simulink model "pwm_controlled_system"  (R2017a)
settings: Solver=FixedStepAuto  StartTime=0.0  StopTime=t_f  FixedStep=1e-6  RelTol=1e-3
values from neighbouring files (symbols this model uses):
  C_ = C    [load_delay.m]
  Ctilde = [Ctilde, zeros(n_Ctilde, s_nds_i + s_nds_o)]    [load_delay.m]    (also in load_pwm_delayed_controller.m = Ctilde(1, 1:2); load_pwm_delayed_pred_controller.m = Ctilde(1, 1:2); load_pwm_pred_controller.m = Ctilde(1:2))
  x0 = [0; 0]    [sim_controlled_system.m]
undefined symbols (not defined in the file or in its folder): A, B, torque_ref, Tpwm_val, Ts_val, Vcc_val
settings Model: Creator=brunolnetto  LastModifiedBy=brunolnetto
settings SolverCC: AlgebraicLoopSolver=LineSearch

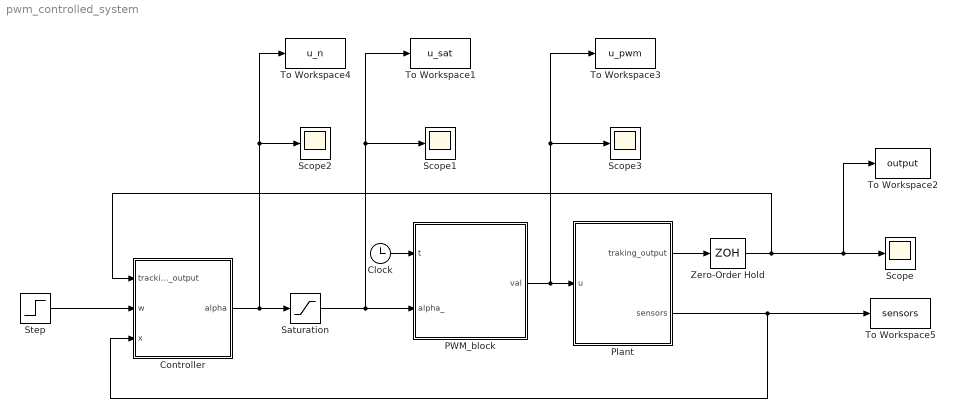
== system pwm_controlled_system ==
  Clock : Clock
  Controller : Subsystem
  PWM_block : MATLAB Function  TreatAsAtomicUnit=on
  Plant : Subsystem
  Saturation : Saturate  UpperLimit=1  LowerLimit=-1
  Scope{,1..3} (4 alike) : Scope
  Step : Step  Time=0  After=torque_ref  SampleTime=Ts_val
  To Workspace1 : ToWorkspace  VariableName=u_sat  SaveFormat=Structure With Time  SampleTime=-1
  To Workspace2 : ToWorkspace  VariableName=output  SaveFormat=Structure With Time  SampleTime=-1
  To Workspace3 : ToWorkspace  VariableName=u_pwm  SaveFormat=Structure With Time  SampleTime=-1
  To Workspace4 : ToWorkspace  VariableName=u_n  SaveFormat=Structure With Time  SampleTime=-1
  To Workspace5 : ToWorkspace  VariableName=sensors  SaveFormat=Structure With Time  SampleTime=-1
  Zero-Order Hold : ZeroOrderHold  SampleTime=-1
  wires:
  Plant/1(traking_output) -> Zero-Order Hold/1
  Plant/2(sensors) -> To Workspace5/1, Controller/3(x)
  Step/1 -> Controller/2(w)
  Controller/1(alpha) -> To Workspace4/1, Scope2/1, Saturation/1
  Saturation/1 -> Scope1/1, To Workspace1/1, PWM_block/2(alpha_)
  PWM_block/1(val) -> Plant/1(u), Scope3/1, To Workspace3/1
  Zero-Order Hold/1 -> To Workspace2/1, Scope/1, Controller/1(tracking_output)
  Clock/1 -> PWM_block/1(t)

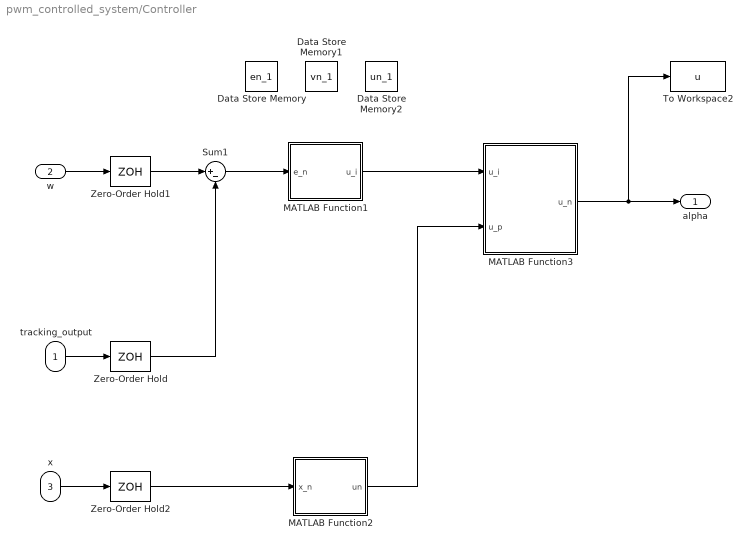
== system pwm_controlled_system/Controller ==
  tracking_output : Inport
  w : Inport  Port=2
  x : Inport  Port=3
  Data Store Memory : DataStoreMemory  DataStoreName=en_1  InitialValue=e0  ShowAdditionalParam=off  OutDataTypeStr=double
  Data Store Memory1 : DataStoreMemory  DataStoreName=vn_1  ShowAdditionalParam=off  OutDataTypeStr=double
  Data Store Memory2 : DataStoreMemory  DataStoreName=un_1  InitialValue=u0  ShowAdditionalParam=off  OutDataTypeStr=double
  MATLAB Function1 : MATLAB Function  TreatAsAtomicUnit=on
  MATLAB Function2 : MATLAB Function  TreatAsAtomicUnit=on
  MATLAB Function3 : MATLAB Function  TreatAsAtomicUnit=on
  Sum1 : Sum  Inputs=|+-
  To Workspace2 : ToWorkspace  VariableName=u  SaveFormat=Structure With Time  SampleTime=-1
  Zero-Order Hold : ZeroOrderHold  SampleTime=Ts_val
  Zero-Order Hold1 : ZeroOrderHold  SampleTime=Ts_val
  Zero-Order Hold2 : ZeroOrderHold  SampleTime=Ts_val
  alpha : Outport
  wires:
  Zero-Order Hold1/1 -> Sum1/1
  tracking_output/1 -> Zero-Order Hold/1
  Zero-Order Hold2/1 -> MATLAB Function2/1(x_n)
  MATLAB Function3/1(u_n) -> To Workspace2/1, alpha/1
  x/1 -> Zero-Order Hold2/1
  Sum1/1 -> MATLAB Function1/1(e_n)
  Zero-Order Hold/1 -> Sum1/2
  w/1 -> Zero-Order Hold1/1
  MATLAB Function2/1(un) -> MATLAB Function3/2(u_p)
  MATLAB Function1/1(u_i) -> MATLAB Function3/1(u_i)

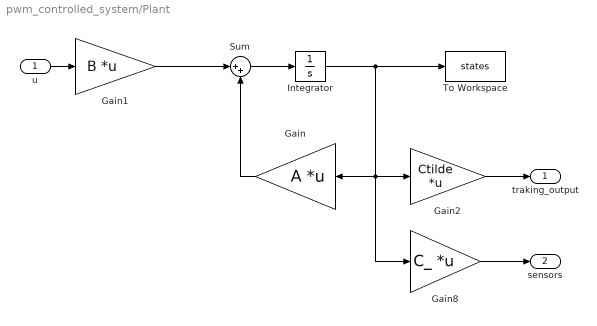
== system pwm_controlled_system/Plant ==
  u : Inport
  Gain : Gain  Gain=A  Multiplication=Matrix(K*u) (u vector)
  Gain1 : Gain  Gain=B  Multiplication=Matrix(K*u) (u vector)
  Gain2 : Gain  Gain=Ctilde  Multiplication=Matrix(K*u) (u vector)
  Gain8 : Gain  Gain=C_  Multiplication=Matrix(K*u) (u vector)
  Integrator : Integrator  InitialCondition=x0
  Sum : Sum  Inputs=|++
  To Workspace : ToWorkspace  VariableName=states  SaveFormat=Structure With Time  SampleTime=-1
  traking_output : Outport
  sensors : Outport  Port=2
  wires:
  Gain8/1 -> sensors/1
  Gain1/1 -> Sum/1
  Integrator/1 -> To Workspace/1, Gain2/1, Gain8/1, Gain/1
  u/1 -> Gain1/1
  Gain/1 -> Sum/2
  Sum/1 -> Integrator/1
  Gain2/1 -> traking_output/1

== matlab function pwm_controlled_system/Controller/MATLAB Function3 ==
  data: u_i input; u_p input; u_n output; en_1 data_store_memory; vn_1 data_store_memory; un_1 data_store_memory
function u_n = integrator(u_i, u_p)
    global un_1;
    
    u_n = u_p + u_i;

    un_1 = u_n;
end

== matlab function pwm_controlled_system/Controller/MATLAB Function1 ==
  data: e_n input; u_i output; en_1 data_store_memory; vn_1 data_store_memory; params parameter
function u_i = integrator(e_n, params)
    global vn_1;
    global en_1;
    
    v_n = vn_1 + en_1 ;
    
    u_i = params.Ki * v_n;
    
    en_1 = e_n;
    vn_1 = v_n;
end

== matlab function pwm_controlled_system/Controller/MATLAB Function2 ==
  data: x_n input; un output; en_1 data_store_memory; vn_1 data_store_memory; params parameter
function un = proportional(x_n, params)
    un = - params.Kp*x_n;
end

== matlab function pwm_controlled_system/PWM_block ==
  data: t input; alpha_ input; val output; Vcc_val parameter; Tpwm_val parameter
function val = pwm_signal(t, alpha_, Vcc_val, Tpwm_val)
    % Static variable
    persistent t0;
    
    if(isempty(t0))
        t0 = 0;
    end
        
    % PWM generation
    if(t == 0)
        t0 = 0;
    end
    
    if(t - t0 > Tpwm_val)
        t0 = t;
    end
    
    % Inner time interval
    t_i = t - t0;
    
    abs_alpha = abs(alpha_);
    sign_alpha = sign(alpha_);
    
    if(t_i <= abs_alpha*Tpwm_val)
        val = sign_alpha*Vcc_val;
    else
        val = 0;
    end
end
